simulink model "inv_rot_pen_RL_cntr_simscape_sldrt_w_recording"  (R2025b)
settings: Solver=ode3  StartTime=0.0  StopTime=30  FixedStep=Ts  RelTol=1e-3
PostLoadFcn:
  | try
  | if isempty(which('ZHAWcbfcn'));
  | callback_fid07124=fopen('ZHAWcbfcn.m','w');
  | [~]=fprintf(callback_fid07124,'%s',get_param([bdroot,'/ Setup SLDRT'],'ClipboardFcn'));
  | [~]=fclose(callback_fid07124);
  | setpref('ZHAW_SLDRT_lib','cb_fcn',which('ZHAWcbfcn'))
  | clear callback_fid07124
  | end
  | catch
  | clear callback_fid07124
  | end
  | Ts=eval(get_param([bdroot,'/ Setup SLDRT'],'Ts'));
InitFcn:
  | Ts=eval(get_param([bdroot,'/ Setup SLDRT'],'Ts'));
StopFcn:
  | myStopFcnAppendInitTime
undefined symbols (not defined in the file): cfg, i_max, K, Kp_i, omega0, param, phi2_disable, phi2_enable, rewardParams, safetyParams, Serial_Port, Standard_Devices, theta0, Tn_i, u_max, X, Y, Z
libraries: sm_lib x19, nesl_utility x6, sldrtlib x3, cstblocks x2, rllib x1, simulink x1
(part 2 of 2)

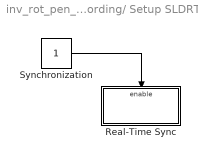
== system inv_rot_pen_RL_cntr_simscape_sldrt_w_recording/ Setup SLDRT ==
  Real-Time Sync : Subsystem
  Synchronization : Constant
  wires:
  Synchronization/1 -> Real-Time Sync/Enable

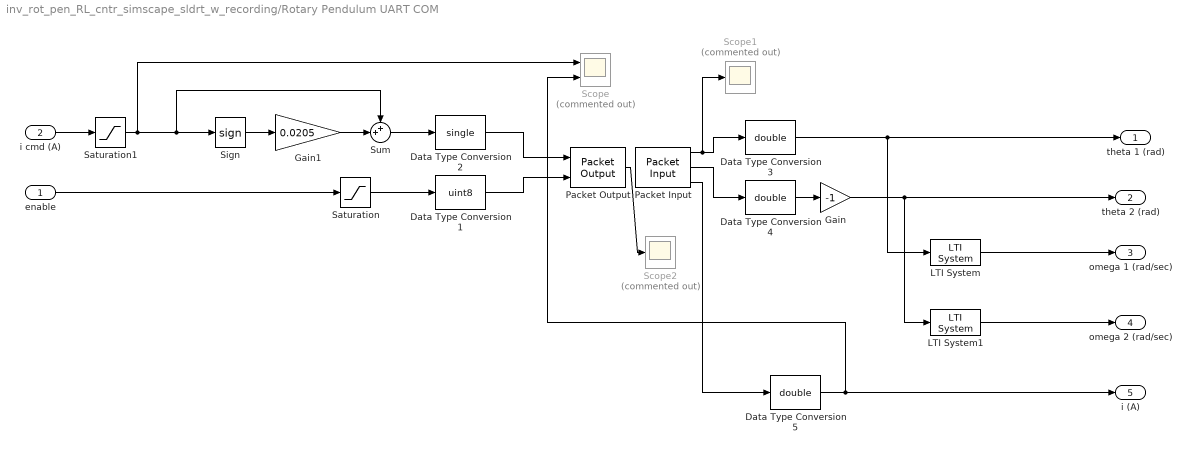
== system inv_rot_pen_RL_cntr_simscape_sldrt_w_recording/Rotary Pendulum UART COM ==
  enable : Inport
  i cmd (A) : Inport  Port=2
  Data Type Conversion1 : DataTypeConversion  OutDataTypeStr=uint8  SaturateOnIntegerOverflow=off  RndMeth=Floor
  Data Type Conversion2 : DataTypeConversion  OutDataTypeStr=single  SaturateOnIntegerOverflow=off  RndMeth=Floor
  Data Type Conversion3 : DataTypeConversion  OutDataTypeStr=double  SaturateOnIntegerOverflow=off  RndMeth=Floor
  Data Type Conversion4 : DataTypeConversion  OutDataTypeStr=double  SaturateOnIntegerOverflow=off  RndMeth=Floor
  Data Type Conversion5 : DataTypeConversion  OutDataTypeStr=double  SaturateOnIntegerOverflow=off  RndMeth=Floor
  Gain : Gain  Gain=-1
  Gain1 : Gain  Gain=0.0205
  LTI System : cstblocks/LTI System  sys=G_diff  IC=[]  PadeOrder=0
  LTI System1 : cstblocks/LTI System  sys=G_diff  IC=[]  PadeOrder=0
  Packet Input : sldrtlib/Packet Input  SampleTime=Ts  MaxMissedTicks=100  ShowMissedTicks=off  YieldWhenWaiting=off  DrvName=Standard_Devices/Serial_Port  DrvAddress=5  DrvOptions=[115200 8 0 0 0 0 0 0]  PacketSize=4 + 4 + 4  DataTypes={'single', 'single', 'single'}  ShowReady=off  ShowError=off  PacketID=1  ByteOrder=1  ShowTimestamp=off
      settings: AttributesFormatString=Serial Port [5]
  Packet Output : sldrtlib/Packet Output  SampleTime=Ts  MaxMissedTicks=100  ShowMissedTicks=on  YieldWhenWaiting=off  DrvName=Standard_Devices/Serial_Port  DrvAddress=5  DrvOptions=[115200 8 0 0 0 0 0 0]  PacketSize=4 + 1  DataTypes={'single', 'uint8'}  ShowReady=off  ShowError=off  PacketID=1  ByteOrder=1  InitialValue=[]  FinalValue=[]
      settings: AttributesFormatString=Serial Port [5]
  Saturation : Saturate  UpperLimit=1.0  LowerLimit=0.0
  Saturation1 : Saturate  UpperLimit=i_max  LowerLimit=-i_max
  Scope : Scope  Commented=on  NumInputPorts=2
      settings: ActiveDisplayYMinimum=-2.5972003042697906  ActiveDisplayYMaximum=2.5919672548770905
  Scope1 : Scope  Commented=on
      settings: ActiveDisplayYMinimum=-1.8320732945576306  ActiveDisplayYMaximum=15.721670583821833
  Scope2 : Scope  Commented=on
      settings: ActiveDisplayYMinimum=-1  ActiveDisplayYMaximum=1  DataLoggingVariableName=ScopeData3
  Sign : Signum
  Sum : Sum  Inputs=++|
  theta 1 (rad) : Outport
  theta 2 (rad) : Outport  Port=2
  omega 1 (rad/sec) : Outport  Port=3
  omega 2 (rad/sec) : Outport  Port=4
  i (A) : Outport  Port=5
  wires:
  Data Type Conversion2/1 -> Packet Output/1
  Packet Input/2 -> Data Type Conversion4/1
  Saturation/1 -> Data Type Conversion1/1
  Packet Input/1 -> Data Type Conversion3/1, Scope1/1
  Data Type Conversion1/1 -> Packet Output/2
  enable/1 -> Saturation/1
  Data Type Conversion3/1 -> LTI System/1, theta 1 (rad)/1
  Data Type Conversion4/1 -> Gain/1
  LTI System/1 -> omega 1 (rad/sec)/1
  LTI System1/1 -> omega 2 (rad/sec)/1
  Gain/1 -> LTI System1/1, theta 2 (rad)/1
  Packet Input/3 -> Data Type Conversion5/1
  Data Type Conversion5/1 -> Scope/2, i (A)/1
  Sign/1 -> Gain1/1
  Gain1/1 -> Sum/2
  i cmd (A)/1 -> Saturation1/1
  Sum/1 -> Data Type Conversion2/1
  Saturation1/1 -> Scope/1, Sum/1, Sign/1
  Packet Output/1 -> Scope2/1

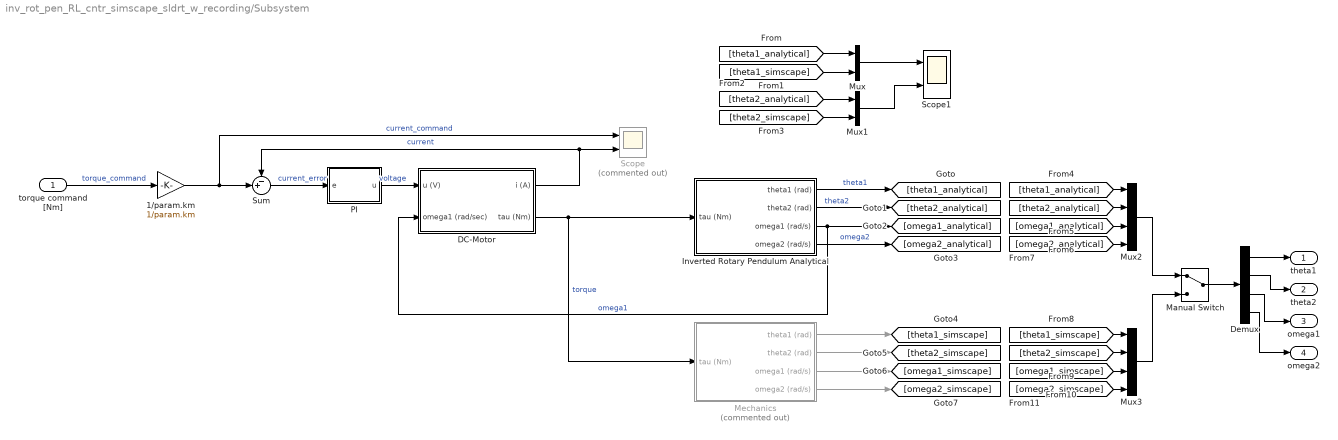
== system inv_rot_pen_RL_cntr_simscape_sldrt_w_recording/Subsystem ==
  torque command [Nm] : Inport
  1/param.km : Gain  Gain=1/param.km
  DC-Motor : Subsystem
  Demux : Demux
  Inverted Rotary Pendulum Analytical : Subsystem
  Manual Switch : ManualSwitch
  Mechanics : Subsystem  Commented=on
  Mux : Mux  Inputs=2
  Mux1 : Mux  Inputs=2
  Mux2 : Mux
  Mux3 : Mux
  PI : Subsystem
  Scope : Scope  Commented=on  NumInputPorts=2
      settings: ActiveDisplayYMinimum=-4.5  ActiveDisplayYMaximum=0.49999999999999989
  Scope1 : Scope  NumInputPorts=2
      settings: ActiveDisplayYMinimum=-0.39852721608277841  ActiveDisplayYMaximum=0.89779085851409868  DataLoggingVariableName=ScopeData6
  Sum : Sum  Inputs=-+|
  theta1 : Outport
  theta2 : Outport  Port=2
  omega1 : Outport  Port=3
  omega2 : Outport  Port=4
  wires:
  Inverted Rotary Pendulum Analytical/3(omega1 (rad/s)) -> [omega1_analytical], DC-Motor/2(omega1 (rad/sec))  "omega1"
  Inverted Rotary Pendulum Analytical/1(theta1 (rad)) -> [theta1_analytical]  "theta1"
  Inverted Rotary Pendulum Analytical/4(omega2 (rad/s)) -> [omega2_analytical]  "omega2"
  Inverted Rotary Pendulum Analytical/2(theta2 (rad)) -> [theta2_analytical]  "theta2"
  PI/1(u) -> DC-Motor/1(u (V))  "voltage"
  DC-Motor/2(tau (Nm)) -> Mechanics/1(tau (Nm)), Inverted Rotary Pendulum Analytical/1(tau (Nm))  "torque"
  1/param.km/1 -> Scope/1, Sum/2  "current_command"
  DC-Motor/1(i (A)) -> Sum/1, Scope/2  "current"
  Sum/1 -> PI/1(e)  "current_error"
  torque command [Nm]/1 -> 1/param.km/1  "torque_command"
  Mux/1 -> Scope1/1
  Mux1/1 -> Scope1/2
  Mechanics/1(theta1 (rad)) -> [theta1_simscape]
  Mechanics/2(theta2 (rad)) -> [theta2_simscape]
  Mechanics/3(omega1 (rad/s)) -> [omega1_simscape]
  Mechanics/4(omega2 (rad/s)) -> [omega2_simscape]
  [theta1_analytical] -> Mux/1
  [theta1_simscape] -> Mux/2
  [theta2_analytical] -> Mux1/1
  [theta2_simscape] -> Mux1/2
  Mux2/1 -> Manual Switch/1
  [theta1_analytical] -> Mux2/1
  [theta2_analytical] -> Mux2/2
  [omega1_analytical] -> Mux2/3
  [omega2_analytical] -> Mux2/4
  [theta1_simscape] -> Mux3/1
  [theta2_simscape] -> Mux3/2
  [omega1_simscape] -> Mux3/3
  [omega2_simscape] -> Mux3/4
  Mux3/1 -> Manual Switch/2
  Demux/1 -> theta1/1
  Demux/2 -> theta2/1
  Demux/3 -> omega1/1
  Demux/4 -> omega2/1
  Manual Switch/1 -> Demux/1

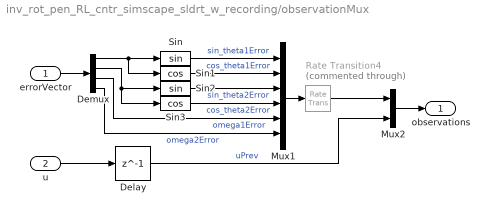
== system inv_rot_pen_RL_cntr_simscape_sldrt_w_recording/observationMux ==
  errorVector : Inport
  u : Inport  Port=2
  Delay : Delay  DelayLength=1
  Demux : Demux
  Mux1 : Mux  Inputs=6
  Mux2 : Mux  Inputs=2
  Rate Transition4 : RateTransition  Commented=through  OutPortSampleTime=cfg.Agent.SampleTime
  Sin : Trigonometry
  Sin1 : Trigonometry  Operator=cos
  Sin2 : Trigonometry
  Sin3 : Trigonometry  Operator=cos
  observations : Outport
  wires:
  Demux/2 -> Sin3/1, Sin2/1
  Sin1/1 -> Mux1/2  "cos_theta1Error"
  Demux/1 -> Sin1/1, Sin/1
  Rate Transition4/1 -> Mux2/1
  Mux1/1 -> Rate Transition4/1
  Sin/1 -> Mux1/1  "sin_theta1Error"
  Sin3/1 -> Mux1/4  "cos_theta2Error"
  errorVector/1 -> Demux/1
  Demux/4 -> Mux1/6  "omega2Error"
  Demux/3 -> Mux1/5  "omega1Error"
  Sin2/1 -> Mux1/3  "sin_theta2Error"
  Mux2/1 -> observations/1
  u/1 -> Delay/1
  Delay/1 -> Mux2/2  "uPrev"

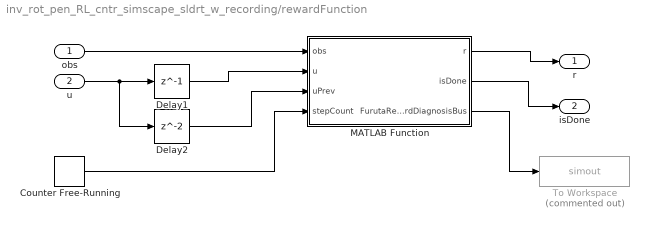
== system inv_rot_pen_RL_cntr_simscape_sldrt_w_recording/rewardFunction ==
  obs : Inport
  u : Inport  Port=2
  Counter Free-Running : simulink/Sources/Counter Free-Running  NumBits=16  tsamp=-1
  Delay1 : Delay  DelayLength=1  SampleTime=cfg.Agent.SampleTime
  Delay2 : Delay  SampleTime=cfg.Agent.SampleTime
  MATLAB Function : MATLAB Function  TreatAsAtomicUnit=on
  To Workspace : ToWorkspace  Commented=on  VariableName=simout  SaveFormat=Timeseries  SampleTime=-1
  r : Outport
  isDone : Outport  Port=2
  wires:
  MATLAB Function/2(isDone) -> isDone/1
  obs/1 -> MATLAB Function/1(obs)
  MATLAB Function/1(r) -> r/1
  u/1 -> Delay2/1, Delay1/1
  Delay2/1 -> MATLAB Function/3(uPrev)
  Delay1/1 -> MATLAB Function/2(u)
  MATLAB Function/3(FurutaRewardDiagnosisBus) -> To Workspace/1
  Counter Free-Running/1 -> MATLAB Function/4(stepCount)

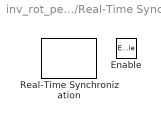
== system inv_rot_pen_RL_cntr_simscape_sldrt_w_recording/ Setup SLDRT/Real-Time Sync ==
  Enable : EnablePort
  Real-Time Synchronization : sldrtlib/Real-Time Synchronization  SampleTime=Ts  MaxMissedTicks=inf  ShowMissedTicks=off  YieldWhenWaiting=off

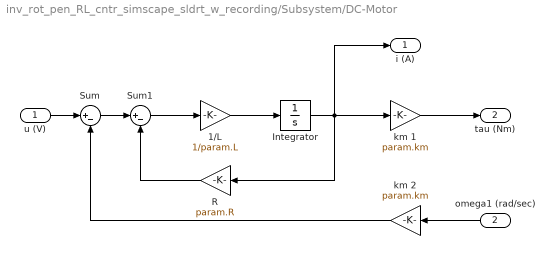
== system inv_rot_pen_RL_cntr_simscape_sldrt_w_recording/Subsystem/DC-Motor ==
  u (V) : Inport
  omega1 (rad/sec) : Inport  Port=2
  1/L : Gain  Gain=1/param.L
  Integrator : Integrator
  R : Gain  Gain=param.R
  Sum : Sum  Inputs=|+-
  Sum1 : Sum  Inputs=|+-
  km 1 : Gain  Gain=param.km
  km 2 : Gain  Gain=param.km
  i (A) : Outport
  tau (Nm) : Outport  Port=2
  wires:
  R/1 -> Sum1/2
  Integrator/1 -> i (A)/1, km 1/1, R/1
  u (V)/1 -> Sum/1
  Sum1/1 -> 1/L/1
  Sum/1 -> Sum1/1
  1/L/1 -> Integrator/1
  omega1 (rad/sec)/1 -> km 2/1
  km 2/1 -> Sum/2
  km 1/1 -> tau (Nm)/1

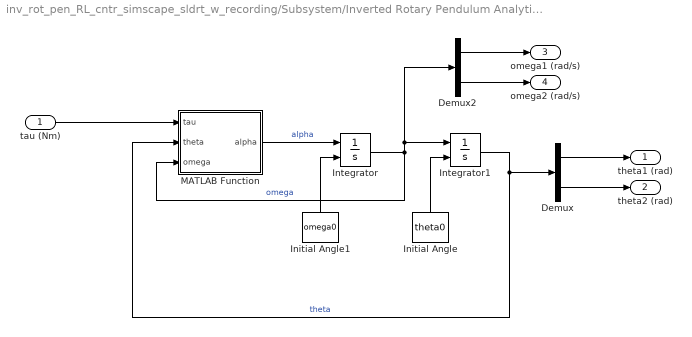
== system inv_rot_pen_RL_cntr_simscape_sldrt_w_recording/Subsystem/Inverted Rotary Pendulum Analytical ==
  tau (Nm) : Inport
  Demux : Demux  Outputs=2
  Demux2 : Demux  Outputs=2
  Initial Angle : Constant  Value=theta0
  Initial Angle1 : Constant  Value=omega0
  Integrator : Integrator  InitialConditionSource=external
  Integrator1 : Integrator  InitialConditionSource=external  InitialCondition=[0.1;0]
  MATLAB Function : MATLAB Function  TreatAsAtomicUnit=on
  theta1 (rad) : Outport
  theta2 (rad) : Outport  Port=2
  omega1 (rad/s) : Outport  Port=3
  omega2 (rad/s) : Outport  Port=4
  wires:
  Demux/2 -> theta2 (rad)/1
  MATLAB Function/1(alpha) -> Integrator/1  "alpha"
  tau (Nm)/1 -> MATLAB Function/1(tau)
  Integrator1/1 -> MATLAB Function/2(theta), Demux/1  "theta"
  Demux/1 -> theta1 (rad)/1
  Integrator/1 -> Demux2/1, Integrator1/1, MATLAB Function/3(omega)  "omega"
  Demux2/1 -> omega1 (rad/s)/1
  Initial Angle/1 -> Integrator1/2
  Demux2/2 -> omega2 (rad/s)/1
  Initial Angle1/1 -> Integrator/2

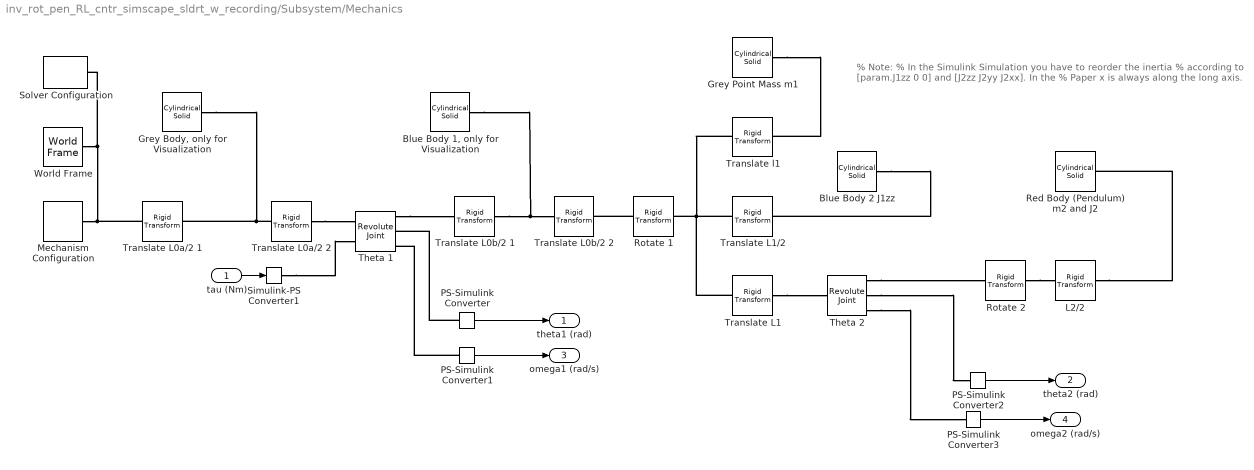
== system inv_rot_pen_RL_cntr_simscape_sldrt_w_recording/Subsystem/Mechanics ==
  note: % Note:
      | % In the Simulink Simulation you have to reorder the inertia
      | % according to [param.J1zz 0 0] and [J2zz J2yy J2xx]. In the
      | % Paper x is always along the long axis.
  tau (Nm) : Inport
  "Blue Body 1, only for Visualization" : sm_lib/Body Elements/Cylindrical Solid  CylinderRadius=param.r0b  CylinderRadiusUnits=m  CylinderLength=param.L0b  CylinderLengthUnits=m  ExportEntireGeometry=off  InertiaType=PointMass  BasedOnType=Density  Density=1000  DensityUnits=kg/m^3  Mass=0  MassUnits=kg  CenterOfMass=[0 0 0]  CenterOfMassUnits=m  MomentsOfInertia=[0 0 0]  MomentsOfInertiaUnits=kg*m^2  ProductsOfInertia=[0 0 0]  ProductsOfInertiaUnits=kg*m^2  GraphicType=FromGeometry  MarkerShape=Sphere  MarkerSize=10  GraphicVisPropType=SimpleVisualProperties  GraphicDiffuseColor=[0.0 0.6 1.0]  GraphicOpacity=1  GraphicSpecularColor=[0.5 0.5 0.5 1.0]  GraphicAmbientColor=[0.15 0.15 0.15 1.0]  GraphicEmissiveColor=[0.0 0.0 0.0 1.0]  GraphicShininess=75  DoExposeReferenceFrame=on  SerializedFrames=<Frames/>
  Blue Body 2 J1zz : sm_lib/Body Elements/Cylindrical Solid  CylinderRadius=param.r1  CylinderRadiusUnits=m  CylinderLength=param.L1  CylinderLengthUnits=m  ExportEntireGeometry=off  InertiaType=Custom  BasedOnType=Density  Density=1000  DensityUnits=kg/m^3  Mass=0  MassUnits=kg  CenterOfMass=[0 0 0]  CenterOfMassUnits=m  MomentsOfInertia=[param.J1zz 0 0]  MomentsOfInertiaUnits=kg*m^2  ProductsOfInertia=[0 0 0]  ProductsOfInertiaUnits=kg*m^2  GraphicType=FromGeometry  MarkerShape=Sphere  MarkerSize=10  GraphicVisPropType=SimpleVisualProperties  GraphicDiffuseColor=[0.0 0.6 1.0]  GraphicOpacity=1  GraphicSpecularColor=[0.5 0.5 0.5 1.0]  GraphicAmbientColor=[0.15 0.15 0.15 1.0]  GraphicEmissiveColor=[0.0 0.0 0.0 1.0]  GraphicShininess=75  DoExposeReferenceFrame=on  SerializedFrames=<Frames/>
  "Grey Body, only for Visualization" : sm_lib/Body Elements/Cylindrical Solid  CylinderRadius=param.r0a  CylinderRadiusUnits=m  CylinderLength=param.L0a  CylinderLengthUnits=m  ExportEntireGeometry=off  InertiaType=PointMass  BasedOnType=Density  Density=1000  DensityUnits=kg/m^3  Mass=0  MassUnits=kg  CenterOfMass=[0 0 0]  CenterOfMassUnits=m  MomentsOfInertia=[0 0 0]  MomentsOfInertiaUnits=kg*m^2  ProductsOfInertia=[0 0 0]  ProductsOfInertiaUnits=kg*m^2  GraphicType=FromGeometry  MarkerShape=Sphere  MarkerSize=10  GraphicVisPropType=SimpleVisualProperties  GraphicDiffuseColor=[0.5 0.5 0.5]  GraphicOpacity=1  GraphicSpecularColor=[0.5 0.5 0.5 1.0]  GraphicAmbientColor=[0.15 0.15 0.15 1.0]  GraphicEmissiveColor=[0.0 0.0 0.0 1.0]  GraphicShininess=75  DoExposeReferenceFrame=on  SerializedFrames=<Frames/>
  Grey Point Mass m1 : sm_lib/Body Elements/Cylindrical Solid  CylinderRadius=1  CylinderRadiusUnits=m  CylinderLength=1  CylinderLengthUnits=m  ExportEntireGeometry=off  InertiaType=PointMass  BasedOnType=Density  Density=1000  DensityUnits=kg/m^3  Mass=param.m1  MassUnits=kg  CenterOfMass=[0 0 0]  CenterOfMassUnits=m  MomentsOfInertia=[1 1 1]  MomentsOfInertiaUnits=kg*m^2  ProductsOfInertia=[0 0 0]  ProductsOfInertiaUnits=kg*m^2  GraphicType=Marker  MarkerShape=Sphere  MarkerSize=10  GraphicVisPropType=SimpleVisualProperties  GraphicDiffuseColor=[0.5 0.5 0.5]  GraphicOpacity=1  GraphicSpecularColor=[0.5 0.5 0.5 1.0]  GraphicAmbientColor=[0.15 0.15 0.15 1.0]  GraphicEmissiveColor=[0.0 0.0 0.0 1.0]  GraphicShininess=75  DoExposeReferenceFrame=on  SerializedFrames=<Frames/>
  L2/2 : sm_lib/Frames and Transforms/Rigid Transform  RotationMethod=None  FollAlignAxisA=+X  BaseAlignAxisA=+Y  FollAlignAxisB=+Y  BaseAlignAxisB=+Z  RotationStandardAxis=+Z  RotationAngle=0  RotationAngleUnits=deg  RotationArbitraryAxis=[0 0 1]  RotationSequenceAxes=FollowerAxes  RotationSequence=ZYX  RotationSequenceAngles=[0 pi/2 0]  RotationSequenceAnglesUnits=rad  RotationMatrix=[1 0 0;0 1 0;0 0 1]  Quaternion=[1 0 0 0]  TranslationMethod=Cartesian  TranslationCartesianOffset=[0 0 param.L2/2]  TranslationCartesianOffsetUnits=m  TranslationStandardAxis=+Z  TranslationStandardOffset=0  TranslationStandardOffsetUnits=m  TranslationROffset=0  TranslationROffsetUnits=m  TranslationThetaOffset=0  TranslationThetaOffsetUnits=deg  TranslationZOffset=0  TranslationZOffsetUnits=m
  Mechanism Configuration : sm_lib/Utilities/Mechanism Configuration  UniformGravity=Constant  GravityVector=[0 0 -param.g]  GravityVectorUnits=m/s^2  LinearizationDelta=0.001  JointModeTransitionNonlinearIterations=2
  PS-Simulink Converter{,1..3} (4 alike) : nesl_utility/PS-Simulink Converter  PhysicalDomain=network_engine_domain  SubClassName=ps_output  LeftPortType=input  RightPortType=output  PseudoPeriodic=off  Frequencies=[]  VectorFormat=inherit  Unit=inherit  AffineConversion=off
  Red Body (Pendulum) m2 and J2 : sm_lib/Body Elements/Cylindrical Solid  CylinderRadius=param.r2  CylinderRadiusUnits=m  CylinderLength=param.L2  CylinderLengthUnits=m  ExportEntireGeometry=off  InertiaType=Custom  BasedOnType=Density  Density=1000  DensityUnits=kg/m^3  Mass=param.m2  MassUnits=kg  CenterOfMass=[0 0 0]  CenterOfMassUnits=m  MomentsOfInertia=[param.J2zz param.J2yy param.J2xx]  MomentsOfInertiaUnits=kg*m^2  ProductsOfInertia=[0 0 0]  ProductsOfInertiaUnits=kg*m^2  GraphicType=FromGeometry  MarkerShape=Sphere  MarkerSize=10  GraphicVisPropType=SimpleVisualProperties  GraphicDiffuseColor=[1.0 0.2 0.2]  GraphicOpacity=1  GraphicSpecularColor=[0.5 0.5 0.5 1.0]  GraphicAmbientColor=[0.15 0.15 0.15 1.0]  GraphicEmissiveColor=[0.0 0.0 0.0 1.0]  GraphicShininess=75  DoExposeReferenceFrame=on  SerializedFrames=<Frames/>
  Rotate 1 : sm_lib/Frames and Transforms/Rigid Transform  RotationMethod=RotationSequence  FollAlignAxisA=+X  BaseAlignAxisA=+Y  FollAlignAxisB=+Y  BaseAlignAxisB=+Z  RotationStandardAxis=+Z  RotationAngle=0  RotationAngleUnits=deg  RotationArbitraryAxis=[0 0 1]  RotationSequenceAxes=FollowerAxes  RotationSequence=ZYX  RotationSequenceAngles=[0 pi/2 0]  RotationSequenceAnglesUnits=rad  RotationMatrix=[1 0 0;0 1 0;0 0 1]  Quaternion=[1 0 0 0]  TranslationMethod=None  TranslationCartesianOffset=[0 0 0]  TranslationCartesianOffsetUnits=m  TranslationStandardAxis=+Z  TranslationStandardOffset=0  TranslationStandardOffsetUnits=m  TranslationROffset=0  TranslationROffsetUnits=m  TranslationThetaOffset=0  TranslationThetaOffsetUnits=deg  TranslationZOffset=0  TranslationZOffsetUnits=m
  Rotate 2 : sm_lib/Frames and Transforms/Rigid Transform  RotationMethod=RotationSequence  FollAlignAxisA=+X  BaseAlignAxisA=+Y  FollAlignAxisB=+Y  BaseAlignAxisB=+Z  RotationStandardAxis=+Z  RotationAngle=0  RotationAngleUnits=deg  RotationArbitraryAxis=[0 0 1]  RotationSequenceAxes=FollowerAxes  RotationSequence=ZYX  RotationSequenceAngles=[0 pi/2 0]  RotationSequenceAnglesUnits=rad  RotationMatrix=[1 0 0;0 1 0;0 0 1]  Quaternion=[1 0 0 0]  TranslationMethod=None  TranslationCartesianOffset=[0 0 0]  TranslationCartesianOffsetUnits=m  TranslationStandardAxis=+Z  TranslationStandardOffset=0  TranslationStandardOffsetUnits=m  TranslationROffset=0  TranslationROffsetUnits=m  TranslationThetaOffset=0  TranslationThetaOffsetUnits=deg  TranslationZOffset=0  TranslationZOffsetUnits=m
  Simulink-PS Converter1 : nesl_utility/Simulink-PS Converter  PhysicalDomain=network_engine_domain  SubClassName=ps_input  LeftPortType=input  RightPortType=output  PseudoPeriodic=off  Frequencies=[]  NoiseDistribution=none  NoiseParameters=[]  Unit=1  AffineConversion=off  FilteringAndDerivatives=provide  SimscapeFilterOrder=1  InputFilterTimeConstant=0.001  UdotUserProvided=0
  Solver Configuration : nesl_utility/Solver Configuration  PhysicalDomain=network_engine_domain  SubClassName=solver  LeftPortType=input  RightPortType=generic  Tones=[]  Harmonics=[]  SimulateNoise=off  Profile=off  UseLocalSampling=off  EnableSwitchedLinearOptims=on  FrequencyDomain=off  UseCCode=off  RelTol=0.001  AbsTol=0.001  MinStep=1e-09  ToWorkspace=off  RevertToSquareIcSolve=off  NumHomotopyIterations=100  PhasorMode=off  PhasorModeNumHarmonics=1  ConsistencySolver=NEWTON_XTOL_AFTER_FTOL  IndexReductionMethod=DerivativeReplacement  DoDC=off  ResidualTolerance=1e-09  ConsistencyTolSource=GLOBAL  ConsistencyAbsTol=0.001  ConsistencyRelTol=0.001  ConsistencyTolFactor=0.001  UseLocalSolver=off  LocalSolverChoice=NE_BACKWARD_EULER_ADVANCER  ResolveIndetEquations=on  FunctionEvalNumThread=1  LocalSolverSampleTime=0.001  DoFixedCost=off  MaxNonlinIter=3  MaxModeIter=2  ComputeImpulses=off  ImpulseIterations=2  LinearAlgebra=auto  LinearAlgebraNumThread=0  EquationFormulation=NE_TIME_EF  DelaysMemoryBudget=1024  AutomaticFiltering=on  FilteringTimeConstant=0.001  PartitionStorageMethod=AS_NEEDED  PartitionMemoryBudget=1024  PartitionMethod=ROBUST  MultibodyUseLocalSolver=off  MultibodyLocalSolverChoice=ODE1  MultibodyLocalSolverSampleTime=0.001
  Theta 1 : sm_lib/Joints/Revolute Joint  JointMode=Normal  CompositeWrenchDir=FollowerOnBase  CompositeWrenchFrame=BaseFrame  SenseConstraintForce=off  SenseConstraintTorque=off  SenseTotalForce=off  SenseTotalTorque=off  PositionTargetSpecify=on  PositionTargetPriority=High  PositionTargetValue=theta0(1)  PositionTargetValueUnits=rad  VelocityTargetSpecify=off  VelocityTargetPriority=High  VelocityTargetValue=0  VelocityTargetValueUnits=deg/s  EquilibriumPosition=0  EquilibriumPositionUnits=rad  SpringStiffness=0  SpringStiffnessUnits=N*m/rad  DampingCoefficient=param.b1  DampingCoefficientUnits=N*m*s/rad  LowerLimitSpecify=off  LowerLimitBound=-90  LowerLimitBoundUnits=deg  LowerLimitStiffness=1e4  LowerLimitStiffnessUnits=N*m/deg  LowerLimitDamping=10  LowerLimitDampingUnits=N*m/(deg/s)  LowerLimitTransitionRegionWidth=0.1  LowerLimitTransitionRegionWidthUnits=deg  UpperLimitSpecify=off  UpperLimitBound=90  UpperLimitBoundUnits=deg  UpperLimitStiffness=1e4  UpperLimitStiffnessUnits=N*m/deg  UpperLimitDamping=10  UpperLimitDampingUnits=N*m/(deg/s)  UpperLimitTransitionRegionWidth=0.1  UpperLimitTransitionRegionWidthUnits=deg  TorqueActuationMode=InputTorque  MotionActuationMode=ComputedMotion  SensePosition=on  SenseVelocity=on  SenseAcceleration=off  SenseTorqueForce=off  SenseLowerLimitTorqueForce=off  SenseUpperLimitTorqueForce=off
  Theta 2 : sm_lib/Joints/Revolute Joint  JointMode=Normal  CompositeWrenchDir=FollowerOnBase  CompositeWrenchFrame=BaseFrame  SenseConstraintForce=off  SenseConstraintTorque=off  SenseTotalForce=off  SenseTotalTorque=off  PositionTargetSpecify=on  PositionTargetPriority=High  PositionTargetValue=theta0(2)  PositionTargetValueUnits=rad  VelocityTargetSpecify=off  VelocityTargetPriority=High  VelocityTargetValue=0  VelocityTargetValueUnits=deg/s  EquilibriumPosition=0  EquilibriumPositionUnits=rad  SpringStiffness=0  SpringStiffnessUnits=N*m/rad  DampingCoefficient=param.b2  DampingCoefficientUnits=N*m*s/rad  LowerLimitSpecify=off  LowerLimitBound=-90  LowerLimitBoundUnits=deg  LowerLimitStiffness=1e4  LowerLimitStiffnessUnits=N*m/deg  LowerLimitDamping=10  LowerLimitDampingUnits=N*m/(deg/s)  LowerLimitTransitionRegionWidth=0.1  LowerLimitTransitionRegionWidthUnits=deg  UpperLimitSpecify=off  UpperLimitBound=90  UpperLimitBoundUnits=deg  UpperLimitStiffness=1e4  UpperLimitStiffnessUnits=N*m/deg  UpperLimitDamping=10  UpperLimitDampingUnits=N*m/(deg/s)  UpperLimitTransitionRegionWidth=0.1  UpperLimitTransitionRegionWidthUnits=deg  TorqueActuationMode=NoTorque  MotionActuationMode=ComputedMotion  SensePosition=on  SenseVelocity=on  SenseAcceleration=off  SenseTorqueForce=off  SenseLowerLimitTorqueForce=off  SenseUpperLimitTorqueForce=off
  Translate L0a/2 1 : sm_lib/Frames and Transforms/Rigid Transform  RotationMethod=None  FollAlignAxisA=+X  BaseAlignAxisA=+Y  FollAlignAxisB=+Y  BaseAlignAxisB=+Z  RotationStandardAxis=+Z  RotationAngle=0  RotationAngleUnits=deg  RotationArbitraryAxis=[0 0 1]  RotationSequenceAxes=FollowerAxes  RotationSequence=ZYX  RotationSequenceAngles=[0 0 0]  RotationSequenceAnglesUnits=rad  RotationMatrix=[1 0 0;0 1 0;0 0 1]  Quaternion=[1 0 0 0]  TranslationMethod=Cartesian  TranslationCartesianOffset=[0 0 param.L0a/2]  TranslationCartesianOffsetUnits=m  TranslationStandardAxis=+Z  TranslationStandardOffset=0  TranslationStandardOffsetUnits=m  TranslationROffset=0  TranslationROffsetUnits=m  TranslationThetaOffset=0  TranslationThetaOffsetUnits=deg  TranslationZOffset=0  TranslationZOffsetUnits=m
  Translate L0a/2 2 : sm_lib/Frames and Transforms/Rigid Transform  RotationMethod=None  FollAlignAxisA=+X  BaseAlignAxisA=+Y  FollAlignAxisB=+Y  BaseAlignAxisB=+Z  RotationStandardAxis=+Z  RotationAngle=0  RotationAngleUnits=deg  RotationArbitraryAxis=[0 0 1]  RotationSequenceAxes=FollowerAxes  RotationSequence=ZYX  RotationSequenceAngles=[0 0 0]  RotationSequenceAnglesUnits=rad  RotationMatrix=[1 0 0;0 1 0;0 0 1]  Quaternion=[1 0 0 0]  TranslationMethod=Cartesian  TranslationCartesianOffset=[0 0 param.L0a/2]  TranslationCartesianOffsetUnits=m  TranslationStandardAxis=+Z  TranslationStandardOffset=0  TranslationStandardOffsetUnits=m  TranslationROffset=0  TranslationROffsetUnits=m  TranslationThetaOffset=0  TranslationThetaOffsetUnits=deg  TranslationZOffset=0  TranslationZOffsetUnits=m
  Translate L0b/2 1 : sm_lib/Frames and Transforms/Rigid Transform  RotationMethod=None  FollAlignAxisA=+X  BaseAlignAxisA=+Y  FollAlignAxisB=+Y  BaseAlignAxisB=+Z  RotationStandardAxis=+Z  RotationAngle=0  RotationAngleUnits=deg  RotationArbitraryAxis=[0 0 1]  RotationSequenceAxes=FollowerAxes  RotationSequence=ZYX  RotationSequenceAngles=[0 0 0]  RotationSequenceAnglesUnits=rad  RotationMatrix=[1 0 0;0 1 0;0 0 1]  Quaternion=[1 0 0 0]  TranslationMethod=Cartesian  TranslationCartesianOffset=[0 0 param.L0b/2]  TranslationCartesianOffsetUnits=m  TranslationStandardAxis=+Z  TranslationStandardOffset=0  TranslationStandardOffsetUnits=m  TranslationROffset=0  TranslationROffsetUnits=m  TranslationThetaOffset=0  TranslationThetaOffsetUnits=deg  TranslationZOffset=0  TranslationZOffsetUnits=m
  Translate L0b/2 2 : sm_lib/Frames and Transforms/Rigid Transform  RotationMethod=None  FollAlignAxisA=+X  BaseAlignAxisA=+Y  FollAlignAxisB=+Y  BaseAlignAxisB=+Z  RotationStandardAxis=+Z  RotationAngle=0  RotationAngleUnits=deg  RotationArbitraryAxis=[0 0 1]  RotationSequenceAxes=FollowerAxes  RotationSequence=ZYX  RotationSequenceAngles=[0 0 0]  RotationSequenceAnglesUnits=rad  RotationMatrix=[1 0 0;0 1 0;0 0 1]  Quaternion=[1 0 0 0]  TranslationMethod=Cartesian  TranslationCartesianOffset=[0 0 param.L0b/2]  TranslationCartesianOffsetUnits=m  TranslationStandardAxis=+Z  TranslationStandardOffset=0  TranslationStandardOffsetUnits=m  TranslationROffset=0  TranslationROffsetUnits=m  TranslationThetaOffset=0  TranslationThetaOffsetUnits=deg  TranslationZOffset=0  TranslationZOffsetUnits=m
  Translate L1 : sm_lib/Frames and Transforms/Rigid Transform  RotationMethod=None  FollAlignAxisA=+X  BaseAlignAxisA=+Y  FollAlignAxisB=+Y  BaseAlignAxisB=+Z  RotationStandardAxis=+Z  RotationAngle=0  RotationAngleUnits=deg  RotationArbitraryAxis=[0 0 1]  RotationSequenceAxes=FollowerAxes  RotationSequence=ZYX  RotationSequenceAngles=[0 0 0]  RotationSequenceAnglesUnits=rad  RotationMatrix=[1 0 0;0 1 0;0 0 1]  Quaternion=[1 0 0 0]  TranslationMethod=Cartesian  TranslationCartesianOffset=[0 0 param.L1]  TranslationCartesianOffsetUnits=m  TranslationStandardAxis=+Z  TranslationStandardOffset=0  TranslationStandardOffsetUnits=m  TranslationROffset=0  TranslationROffsetUnits=m  TranslationThetaOffset=0  TranslationThetaOffsetUnits=deg  TranslationZOffset=0  TranslationZOffsetUnits=m
  Translate L1/2 : sm_lib/Frames and Transforms/Rigid Transform  RotationMethod=None  FollAlignAxisA=+X  BaseAlignAxisA=+Y  FollAlignAxisB=+Y  BaseAlignAxisB=+Z  RotationStandardAxis=+Z  RotationAngle=0  RotationAngleUnits=deg  RotationArbitraryAxis=[0 0 1]  RotationSequenceAxes=FollowerAxes  RotationSequence=ZYX  RotationSequenceAngles=[0 0 0]  RotationSequenceAnglesUnits=rad  RotationMatrix=[1 0 0;0 1 0;0 0 1]  Quaternion=[1 0 0 0]  TranslationMethod=Cartesian  TranslationCartesianOffset=[0 0 param.L1/2]  TranslationCartesianOffsetUnits=m  TranslationStandardAxis=+Z  TranslationStandardOffset=0  TranslationStandardOffsetUnits=m  TranslationROffset=0  TranslationROffsetUnits=m  TranslationThetaOffset=0  TranslationThetaOffsetUnits=deg  TranslationZOffset=0  TranslationZOffsetUnits=m
  Translate l1 : sm_lib/Frames and Transforms/Rigid Transform  RotationMethod=None  FollAlignAxisA=+X  BaseAlignAxisA=+Y  FollAlignAxisB=+Y  BaseAlignAxisB=+Z  RotationStandardAxis=+Z  RotationAngle=0  RotationAngleUnits=deg  RotationArbitraryAxis=[0 0 1]  RotationSequenceAxes=FollowerAxes  RotationSequence=ZYX  RotationSequenceAngles=[0 0 0]  RotationSequenceAnglesUnits=rad  RotationMatrix=[1 0 0;0 1 0;0 0 1]  Quaternion=[1 0 0 0]  TranslationMethod=Cartesian  TranslationCartesianOffset=[0 0 param.l1]  TranslationCartesianOffsetUnits=m  TranslationStandardAxis=+Z  TranslationStandardOffset=0  TranslationStandardOffsetUnits=m  TranslationROffset=0  TranslationROffsetUnits=m  TranslationThetaOffset=0  TranslationThetaOffsetUnits=deg  TranslationZOffset=0  TranslationZOffsetUnits=m
  World Frame : sm_lib/Frames and Transforms/World Frame
  theta1 (rad) : Outport
  theta2 (rad) : Outport  Port=2
  omega1 (rad/s) : Outport  Port=3
  omega2 (rad/s) : Outport  Port=4
  wires:
  PS-Simulink Converter2/1 -> theta2 (rad)/1
  PS-Simulink Converter1/1 -> omega1 (rad/s)/1
  PS-Simulink Converter3/1 -> omega2 (rad/s)/1
  tau (Nm)/1 -> Simulink-PS Converter1/1
  PS-Simulink Converter/1 -> theta1 (rad)/1
  connections:
  PS-Simulink Converter1/LConn1 -- Theta 1/RConn3
  Rotate 1/LConn1 -- Translate L0b/2 2/RConn1
  Translate L1/RConn1 -- Theta 2/LConn1
  World Frame/RConn1 -- Translate L0a/2 1/LConn1 -- Mechanism Configuration/RConn1 -- Solver Configuration/RConn1
  Rotate 2/RConn1 -- L2/2/LConn1
  Translate L0a/2 2/LConn1 -- "Grey Body, only for Visualization"/RConn1 -- Translate L0a/2 1/RConn1
  Theta 2/RConn3 -- PS-Simulink Converter3/LConn1
  Theta 2/RConn2 -- PS-Simulink Converter2/LConn1
  Translate L0b/2 1/RConn1 -- "Blue Body 1, only for Visualization"/RConn1 -- Translate L0b/2 2/LConn1
  Theta 1/RConn1 -- Translate L0b/2 1/LConn1
  PS-Simulink Converter/LConn1 -- Theta 1/RConn2
  Translate l1/LConn1 -- Translate L1/2/LConn1 -- Translate L1/LConn1 -- Rotate 1/RConn1
  Blue Body 2 J1zz/RConn1 -- Translate L1/2/RConn1
  Simulink-PS Converter1/RConn1 -- Theta 1/LConn2
  Translate L0a/2 2/RConn1 -- Theta 1/LConn1
  Theta 2/RConn1 -- Rotate 2/LConn1
  Grey Point Mass m1/RConn1 -- Translate l1/RConn1
  L2/2/RConn1 -- Red Body (Pendulum) m2 and J2/RConn1

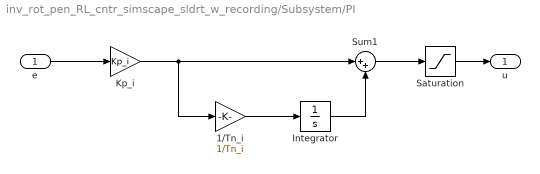
== system inv_rot_pen_RL_cntr_simscape_sldrt_w_recording/Subsystem/PI ==
  e : Inport
  1/Tn_i : Gain  Gain=1/Tn_i
  Integrator : Integrator  UpperSaturationLimit=i_max  LowerSaturationLimit=-i_max
  Kp_i : Gain  Gain=Kp_i
  Saturation : Saturate  UpperLimit=u_max  LowerLimit=-u_max
  Sum1 : Sum  Inputs=|++
  u : Outport
  wires:
  Integrator/1 -> Sum1/2
  Sum1/1 -> Saturation/1
  Kp_i/1 -> Sum1/1, 1/Tn_i/1
  1/Tn_i/1 -> Integrator/1
  e/1 -> Kp_i/1
  Saturation/1 -> u/1

== matlab function inv_rot_pen_RL_cntr_simscape_sldrt_w_recording/Subsystem/Inverted Rotary Pendulum Analytical/MATLAB Function ==
  data: tau input size=1; alpha output size=[2,1]; theta input size=[2,1]; omega input size=[2,1]; param parameter
function alpha = fcn(tau, theta, omega, param)

    % M(q) * qdd + C(q,qdot) * qdot + G(q) + D * qdot = tau
    [M, C, G, D] = calculate_dynamics_furuta(theta, omega, param);
    alpha = M \ ( [tau; 0] - (C + D) * omega - G );

end

== matlab function inv_rot_pen_RL_cntr_simscape_sldrt_w_recording/rewardFunction/MATLAB Function ==
  data: obs input; u input; uPrev input; stepCount input; rewardParams parameter; r output; isDone output; safetyParams parameter; FurutaRewardDiagnosisBus output Bus: FurutaRewardDiagnosisBus
function [r, isDone, FurutaRewardDiagnosisBus] = fcn(obs, u, uPrev, stepCount, rewardParams, safetyParams)
% params declared as block Parameter via Ports & Data Manager
[r, isDone, FurutaRewardDiagnosisBus] = rewardFcnFuruta(obs, u, uPrev, stepCount, rewardParams, safetyParams);
end

== matlab function inv_rot_pen_RL_cntr_simscape_sldrt_w_recording/Enable in Bounds Once ==
  settings: updateMethod=DISCRETE  sampleTime=Ts
  data: phi2 input; Enable output; phi2_enable parameter; phi2_disable parameter
function Enable = fcn(phi2, phi2_enable, phi2_disable)
% One-shot hysteresis switch:
%  - Activates when   |phi2| <= phi2_enable   (only if never activated before)
%  - Deactivates when |phi2| >= phi2_disable  (after activation)
%  - Cannot be activated again once deactivated
%
% Inputs:
%   phi2         current angle in radians
%   phi2_enable  activation threshold (inner) in radians
%   phi2_disable deactivation threshold (outer) in radians
%
% Output:
%   Enable = 1 when active, 0 when inactive (locked after first deactivate)

    persistent active_state has_been_enabled_once
    if isempty(active_state)
        active_state = false;
        has_been_enabled_once = false;
    end

    % Normalize thresholds: ensure inner <= outer (bulletproofing #1)
    if phi2_disable < phi2_enable
        tmp = phi2_enable;
        phi2_enable = phi2_disable;
        phi2_disable = tmp;
    end

    if ~has_been_enabled_once
        % Enable once when inside the inner band (bulletproofing #2: inclusive)
        if abs(phi2) <= phi2_enable
            active_state = true;

        % After activation, disable once when outside the outer band (inclusive)
        elseif active_state && abs(phi2) >= phi2_disable
            active_state = false;
            has_been_enabled_once = true;   % lock out reactivation
        end
    end

    Enable = double(active_state);
end
